simulink model "ins_anello_v2"  (R2026a)
settings: Solver=FixedStepAuto
settings Model: Creator=Usuario  LastModifiedBy=Edison Altamirano

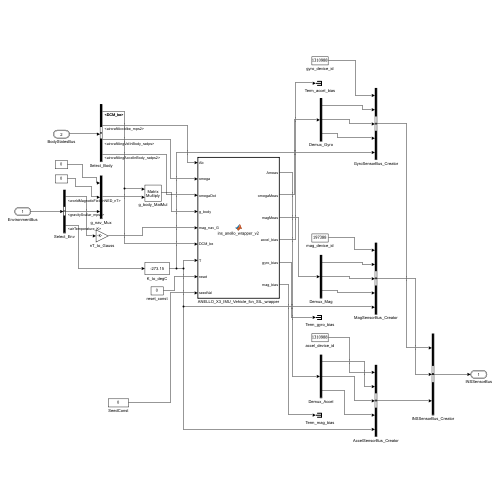
[thumbnail: Simulink's stored preview of the top-level diagram]
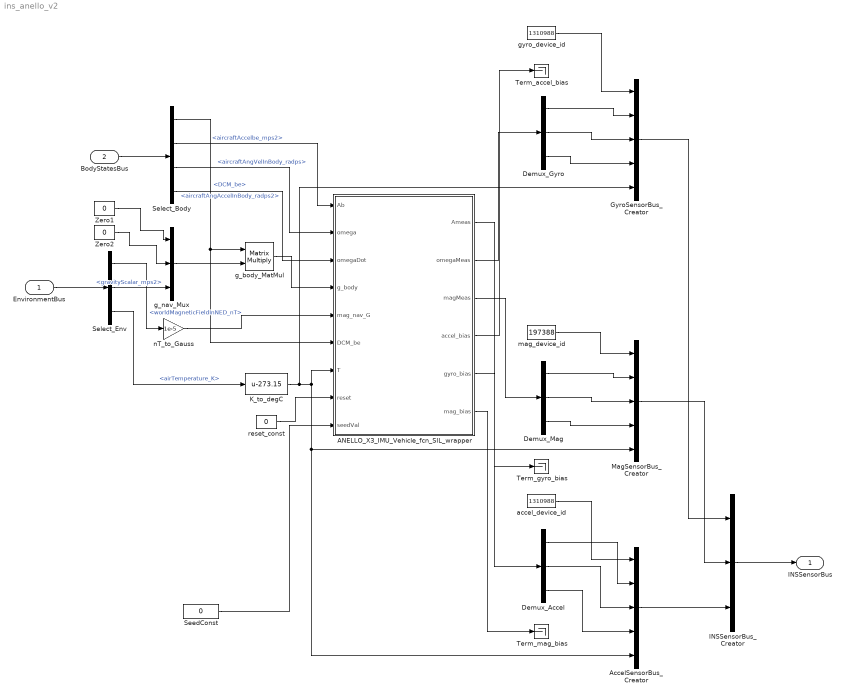
== system ins_anello_v2 ==
  EnvironmentBus : Inport  OutDataTypeStr=Bus: EnvironmentBus
  BodyStatesBus : Inport  Port=2  OutDataTypeStr=Bus: BodyStateBus
  ANELLO_X3_IMU_Vehicle_fcn_SIL_wrapper : MATLAB Function  TreatAsAtomicUnit=on
  AccelSensorBus_Creator : BusCreator  Inputs=5  OutDataTypeStr=Bus: AccelSensorBus
  Demux_Accel : Demux  Outputs=3
  Demux_Gyro : Demux  Outputs=3
  Demux_Mag : Demux  Outputs=3
  GyroSensorBus_Creator : BusCreator  Inputs=5  OutDataTypeStr=Bus: GyroSensorBus
  INSSensorBus_Creator : BusCreator  Inputs=3  OutDataTypeStr=Bus: INSSensorBus
  K_to_degC : Bias  Bias=-273.15  SaturateOnIntegerOverflow=off
  MagSensorBus_Creator : BusCreator  Inputs=5  OutDataTypeStr=Bus: MagSensorBus
  SeedConst : Constant  Value=0
  Select_Body : BusSelector  OutputSignals=DCM_be,aircraftAccelbe_mps2,aircraftAngVelInBody_radps,aircraftAngAccelInBody_radps2
  Select_Env : BusSelector  OutputSignals=EarthEnvironment.worldMagneticFieldInNED_nT,EarthEnvironment.gravityScalar_mps2,AirEnvironment.airTemperature_K
  Term_accel_bias : Terminator
  Term_gyro_bias : Terminator
  Term_mag_bias : Terminator
  Zero1 : Constant  Value=0
  Zero2 : Constant  Value=0
  accel_device_id : Constant  Value=1310988
  g_body_MatMul : Product  Multiplication=Matrix(*)
  g_nav_Mux : Mux  Inputs=3
  gyro_device_id : Constant  Value=1310988
  mag_device_id : Constant  Value=197388
  nT_to_Gauss : Gain  Gain=1e-5
  reset_const : Constant  Value=0
  INSSensorBus : Outport  OutDataTypeStr=Bus: INSSensorBus
  wires:
  EnvironmentBus/1 -> Select_Env/1
  Select_Body/1 -> ANELLO_X3_IMU_Vehicle_fcn_SIL_wrapper/6(DCM_be), g_body_MatMul/1  "<DCM_be>"
  Select_Env/2 -> g_nav_Mux/3  "<gravityScalar_mps2>"
  BodyStatesBus/1 -> Select_Body/1
  Select_Env/3 -> K_to_degC/1  "<airTemperature_K>"
  Zero1/1 -> g_nav_Mux/1
  Select_Env/1 -> nT_to_Gauss/1  "<worldMagneticFieldInNED_nT>"
  Zero2/1 -> g_nav_Mux/2
  INSSensorBus_Creator/1 -> INSSensorBus/1
  Select_Body/2 -> ANELLO_X3_IMU_Vehicle_fcn_SIL_wrapper/1(Ab)  "<aircraftAccelbe_mps2>"
  Select_Body/3 -> ANELLO_X3_IMU_Vehicle_fcn_SIL_wrapper/2(omega)  "<aircraftAngVelInBody_radps>"
  Select_Body/4 -> ANELLO_X3_IMU_Vehicle_fcn_SIL_wrapper/3(omegaDot)  "<aircraftAngAccelInBody_radps2>"
  GyroSensorBus_Creator/1 -> INSSensorBus_Creator/1
  g_nav_Mux/1 -> g_body_MatMul/2
  nT_to_Gauss/1 -> ANELLO_X3_IMU_Vehicle_fcn_SIL_wrapper/5(mag_nav_G)
  MagSensorBus_Creator/1 -> INSSensorBus_Creator/2
  g_body_MatMul/1 -> ANELLO_X3_IMU_Vehicle_fcn_SIL_wrapper/4(g_body)
  K_to_degC/1 -> MagSensorBus_Creator/5, AccelSensorBus_Creator/5, ANELLO_X3_IMU_Vehicle_fcn_SIL_wrapper/7(T), GyroSensorBus_Creator/5
  reset_const/1 -> ANELLO_X3_IMU_Vehicle_fcn_SIL_wrapper/8(reset)
  ANELLO_X3_IMU_Vehicle_fcn_SIL_wrapper/1(Ameas) -> Demux_Accel/1
  ANELLO_X3_IMU_Vehicle_fcn_SIL_wrapper/2(omegaMeas) -> Demux_Gyro/1
  Demux_Accel/1 -> AccelSensorBus_Creator/2
  ANELLO_X3_IMU_Vehicle_fcn_SIL_wrapper/3(magMeas) -> Demux_Mag/1
  Demux_Gyro/1 -> GyroSensorBus_Creator/2
  ANELLO_X3_IMU_Vehicle_fcn_SIL_wrapper/4(accel_bias) -> Term_accel_bias/1
  ANELLO_X3_IMU_Vehicle_fcn_SIL_wrapper/5(gyro_bias) -> Term_gyro_bias/1
  ANELLO_X3_IMU_Vehicle_fcn_SIL_wrapper/6(mag_bias) -> Term_mag_bias/1
  Demux_Mag/3 -> MagSensorBus_Creator/4
  gyro_device_id/1 -> GyroSensorBus_Creator/1
  Demux_Gyro/2 -> GyroSensorBus_Creator/3
  Demux_Gyro/3 -> GyroSensorBus_Creator/4
  Demux_Mag/1 -> MagSensorBus_Creator/2
  mag_device_id/1 -> MagSensorBus_Creator/1
  Demux_Mag/2 -> MagSensorBus_Creator/3
  accel_device_id/1 -> AccelSensorBus_Creator/1
  Demux_Accel/2 -> AccelSensorBus_Creator/3
  Demux_Accel/3 -> AccelSensorBus_Creator/4
  AccelSensorBus_Creator/1 -> INSSensorBus_Creator/3
  SeedConst/1 -> ANELLO_X3_IMU_Vehicle_fcn_SIL_wrapper/9(seedVal)

== matlab function ins_anello_v2/ANELLO_X3_IMU_Vehicle_fcn_SIL_wrapper ==
  data: Ab input; Ameas output; omega input; omegaDot input; g_body input; mag_nav_G input; DCM_be input; T input; reset input; omegaMeas output; magMeas output; accel_bias output; gyro_bias output; mag_bias output; seedVal input
function [Ameas, omegaMeas, magMeas, accel_bias, gyro_bias, mag_bias] = ...
         ins_anello_wrapper_v2(Ab, omega, omegaDot, g_body, mag_nav_G, DCM_be, T, reset, seedVal)
%#codegen
R_bn_vec = DCM_be(:);
[Ameas, omegaMeas, magMeas, accel_bias, gyro_bias, mag_bias] = ...
    ANELLO_X3_IMU_Vehicle_fcn_SIL_v2(Ab, omega, omegaDot, g_body, mag_nav_G, R_bn_vec, T, reset, seedVal);
end
